simulink model "soc_WLAN_fpga"  (R2024b)
settings: Solver=FixedStepDiscrete  StartTime=0.0  StopTime=stopTime  RelTol=1e-3
PreLoadFcn:
  | addpath(fullfile(matlabroot,'toolbox','whdl','whdlexamples','whdlexamples'));
InitFcn:
  | addpath(fullfile(matlabroot,'toolbox','whdl','whdlexamples','whdlexamples'));
model workspace (MAT data in the model file):
  socvcb : containers.Map (value not decoded)
undefined symbols (not defined in the file): Add, bitRatePerOfdmSym, chanBW, coe, cpLen, dataUpsampleFactor, DelayValMaxNsdMinusLastPilotSc, DescramblerInitialSeed, designMultirateFIR, fftLen, filterLatency, filterUpsampleFactor, Fs, Hd, HT_MFMCS0, HT_MFMCS1, HT_MFMCS2, HT_MFMCS3, HT_MFMCS4, HT_MFMCS5, HT_MFMCS6, HT_MFMCS7, HTUnUsedScInd, inputSamplingRate, interp_coeff, maxPilotRefCounterVale, maxPilotsRef, maxPilotsRefNonHT, Ncol_HT, Ncol_NonHT, noDataSubCarriers, Non_HTMCS0, Non_HTMCS1, Non_HTMCS2, Non_HTMCS3, Non_HTMCS4, Non_HTMCS5, Non_HTMCS6, Non_HTMCS7, Nrow_HT, Nrow_NonHT, numDSC_HT, numDSC_HT_vhtSigB, numDSC_NonHT, numDscHT, numDscNonHT, numOfBitsPerOFDMSym, numOfDataBitsPerOFDMSym, numPilots, numScHT, numSCS_HT, numSCS_NonHT, pnSeq, QAM, rxDownsampleFactor, secondPIdx_HT, secondPIdx_NonHT, Shift, VHTMCS0, VHTMCS1 ... (+7)
libraries: hdlsllib x267, simulink x210, dspsigops x22, whdlutilities x10, whdlmod x9, dsphdlfiltering2 x5, dsphdlmathfun2 x4, whdledac x3, hwlogicconnlib x2, commhdlcrc x2, dsphdlsigops2 x2
(part 5 of 14)

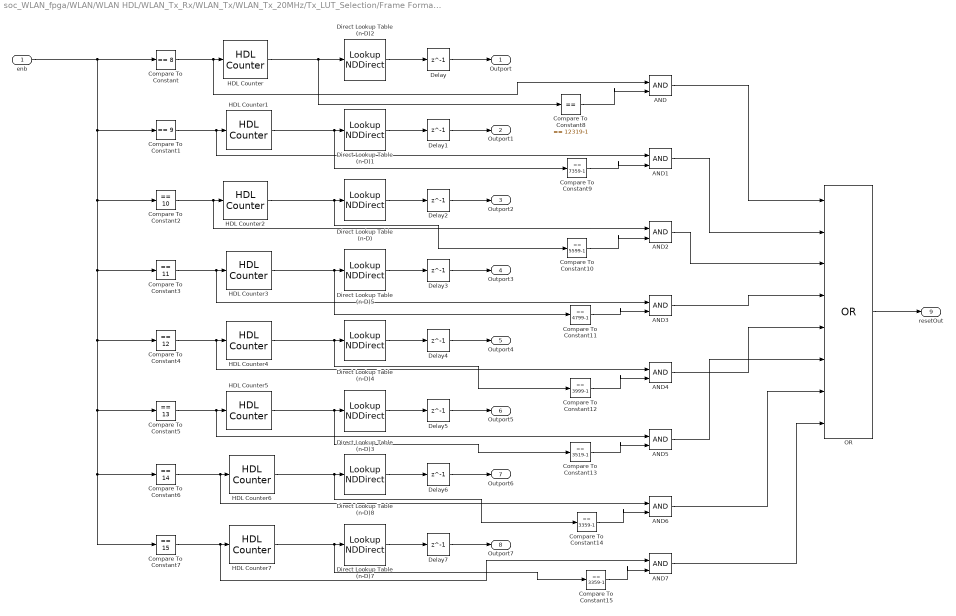
== system soc_WLAN_fpga/WLAN/WLAN HDL/WLAN_Tx_Rx/WLAN_Tx/WLAN_Tx_20MHz/Tx_LUT_Selection/Frame Format 1 ==
  enb : Inport
  AND{,1..7} (8 alike) : Logic  IconShape=distinctive  AllPortsSameDT=off  OutDataTypeStr=boolean
  Compare To Constant : simulink/Logic and Bit Operations/Compare To Constant  relop===  const=8  OutDataTypeStr=boolean
  Compare To Constant1 : simulink/Logic and Bit Operations/Compare To Constant  relop===  const=9  OutDataTypeStr=boolean
  Compare To Constant10 : simulink/Logic and Bit Operations/Compare To Constant  relop===  const=5599-1  OutDataTypeStr=boolean
  Compare To Constant11 : simulink/Logic and Bit Operations/Compare To Constant  relop===  const=4799-1  OutDataTypeStr=boolean
  Compare To Constant12 : simulink/Logic and Bit Operations/Compare To Constant  relop===  const=3999-1  OutDataTypeStr=boolean
  Compare To Constant13 : simulink/Logic and Bit Operations/Compare To Constant  relop===  const=3519-1  OutDataTypeStr=boolean
  Compare To Constant14 : simulink/Logic and Bit Operations/Compare To Constant  relop===  const=3359-1  OutDataTypeStr=boolean
  Compare To Constant15 : simulink/Logic and Bit Operations/Compare To Constant  relop===  const=3359-1  OutDataTypeStr=boolean
  Compare To Constant2 : simulink/Logic and Bit Operations/Compare To Constant  relop===  const=10  OutDataTypeStr=boolean
  Compare To Constant3 : simulink/Logic and Bit Operations/Compare To Constant  relop===  const=11  OutDataTypeStr=boolean
  Compare To Constant4 : simulink/Logic and Bit Operations/Compare To Constant  relop===  const=12  OutDataTypeStr=boolean
  Compare To Constant5 : simulink/Logic and Bit Operations/Compare To Constant  relop===  const=13  OutDataTypeStr=boolean
  Compare To Constant6 : simulink/Logic and Bit Operations/Compare To Constant  relop===  const=14  OutDataTypeStr=boolean
  Compare To Constant7 : simulink/Logic and Bit Operations/Compare To Constant  relop===  const=15  OutDataTypeStr=boolean
  Compare To Constant8 : simulink/Logic and Bit Operations/Compare To Constant  relop===  const=12319-1  OutDataTypeStr=boolean
  Compare To Constant9 : simulink/Logic and Bit Operations/Compare To Constant  relop===  const=7359-1  OutDataTypeStr=boolean
  Delay{,1..7} (8 alike) : Delay  DelayLength=1
  Direct Lookup Table (n-D) : LookupNDDirect  NumberOfTableDimensions=1  Table=HT_MFMCS2
  Direct Lookup Table (n-D)1 : LookupNDDirect  NumberOfTableDimensions=1  Table=HT_MFMCS1
  Direct Lookup Table (n-D)2 : LookupNDDirect  NumberOfTableDimensions=1  Table=HT_MFMCS0
  Direct Lookup Table (n-D)3 : LookupNDDirect  NumberOfTableDimensions=1  Table=HT_MFMCS5
  Direct Lookup Table (n-D)4 : LookupNDDirect  NumberOfTableDimensions=1  Table=HT_MFMCS4
  Direct Lookup Table (n-D)5 : LookupNDDirect  NumberOfTableDimensions=1  Table=HT_MFMCS3
  Direct Lookup Table (n-D)7 : LookupNDDirect  NumberOfTableDimensions=1  Table=HT_MFMCS7
  Direct Lookup Table (n-D)8 : LookupNDDirect  NumberOfTableDimensions=1  Table=HT_MFMCS6
  HDL Counter : hdlsllib/Sources/HDL Counter  CountType=Count limited  CountInit=0  CountStep=1  CountMax=12319  CountFromType=Initial value  CountFrom=0  CountResetPort=off  CountLoadPort=off  CountEnbPort=on  CountDirPort=off  CountHitOutputPort=off  CountDataType=Unsigned  CountWordLen=16  CountFracLen=0  CountSampTime=1
  HDL Counter1 : hdlsllib/Sources/HDL Counter  CountType=Count limited  CountInit=0  CountStep=1  CountMax=7359  CountFromType=Initial value  CountFrom=0  CountResetPort=off  CountLoadPort=off  CountEnbPort=on  CountDirPort=off  CountHitOutputPort=off  CountDataType=Unsigned  CountWordLen=16  CountFracLen=0  CountSampTime=1
  HDL Counter2 : hdlsllib/Sources/HDL Counter  CountType=Count limited  CountInit=0  CountStep=1  CountMax=5599  CountFromType=Initial value  CountFrom=0  CountResetPort=off  CountLoadPort=off  CountEnbPort=on  CountDirPort=off  CountHitOutputPort=off  CountDataType=Unsigned  CountWordLen=16  CountFracLen=0  CountSampTime=1
  HDL Counter3 : hdlsllib/Sources/HDL Counter  CountType=Count limited  CountInit=0  CountStep=1  CountMax=4799  CountFromType=Initial value  CountFrom=0  CountResetPort=off  CountLoadPort=off  CountEnbPort=on  CountDirPort=off  CountHitOutputPort=off  CountDataType=Unsigned  CountWordLen=16  CountFracLen=0  CountSampTime=1
  HDL Counter4 : hdlsllib/Sources/HDL Counter  CountType=Count limited  CountInit=0  CountStep=1  CountMax=3999  CountFromType=Initial value  CountFrom=0  CountResetPort=off  CountLoadPort=off  CountEnbPort=on  CountDirPort=off  CountHitOutputPort=off  CountDataType=Unsigned  CountWordLen=16  CountFracLen=0  CountSampTime=1
  HDL Counter5 : hdlsllib/Sources/HDL Counter  CountType=Count limited  CountInit=0  CountStep=1  CountMax=3519  CountFromType=Initial value  CountFrom=0  CountResetPort=off  CountLoadPort=off  CountEnbPort=on  CountDirPort=off  CountHitOutputPort=off  CountDataType=Unsigned  CountWordLen=16  CountFracLen=0  CountSampTime=1
  HDL Counter6 : hdlsllib/Sources/HDL Counter  CountType=Count limited  CountInit=0  CountStep=1  CountMax=3359  CountFromType=Initial value  CountFrom=0  CountResetPort=off  CountLoadPort=off  CountEnbPort=on  CountDirPort=off  CountHitOutputPort=off  CountDataType=Unsigned  CountWordLen=16  CountFracLen=0  CountSampTime=1
  HDL Counter7 : hdlsllib/Sources/HDL Counter  CountType=Count limited  CountInit=0  CountStep=1  CountMax=3359  CountFromType=Initial value  CountFrom=0  CountResetPort=off  CountLoadPort=off  CountEnbPort=on  CountDirPort=off  CountHitOutputPort=off  CountDataType=Unsigned  CountWordLen=16  CountFracLen=0  CountSampTime=1
  OR : Logic  Operator=OR  Inputs=8  IconShape=distinctive  AllPortsSameDT=off  OutDataTypeStr=boolean
  Outport : Outport
  Outport1 : Outport  Port=2
  Outport2 : Outport  Port=3
  Outport3 : Outport  Port=4
  Outport4 : Outport  Port=5
  Outport5 : Outport  Port=6
  Outport6 : Outport  Port=7
  Outport7 : Outport  Port=8
  resetOut : Outport  Port=9
  wires:
  Delay2/1 -> Outport2/1
  Delay/1 -> Outport/1
  Direct Lookup Table (n-D)1/1 -> Delay1/1
  Direct Lookup Table (n-D)/1 -> Delay2/1
  Direct Lookup Table (n-D)2/1 -> Delay/1
  Delay1/1 -> Outport1/1
  Delay4/1 -> Outport4/1
  Delay5/1 -> Outport5/1
  Direct Lookup Table (n-D)5/1 -> Delay3/1
  Direct Lookup Table (n-D)4/1 -> Delay4/1
  Direct Lookup Table (n-D)3/1 -> Delay5/1
  Delay3/1 -> Outport3/1
  Delay7/1 -> Outport7/1
  Direct Lookup Table (n-D)8/1 -> Delay6/1
  Direct Lookup Table (n-D)7/1 -> Delay7/1
  Delay6/1 -> Outport6/1
  Compare To Constant/1 -> AND/1, HDL Counter/1
  HDL Counter/1 -> Direct Lookup Table (n-D)2/1, Compare To Constant8/1
  HDL Counter1/1 -> Compare To Constant9/1, Direct Lookup Table (n-D)1/1
  Compare To Constant1/1 -> AND1/1, HDL Counter1/1
  HDL Counter2/1 -> Compare To Constant10/1, Direct Lookup Table (n-D)/1
  Compare To Constant2/1 -> AND2/1, HDL Counter2/1
  HDL Counter3/1 -> Compare To Constant11/1, Direct Lookup Table (n-D)5/1
  Compare To Constant3/1 -> AND3/1, HDL Counter3/1
  HDL Counter4/1 -> Compare To Constant12/1, Direct Lookup Table (n-D)4/1
  Compare To Constant4/1 -> AND4/1, HDL Counter4/1
  HDL Counter5/1 -> Compare To Constant13/1, Direct Lookup Table (n-D)3/1
  Compare To Constant5/1 -> AND5/1, HDL Counter5/1
  HDL Counter6/1 -> Compare To Constant14/1, Direct Lookup Table (n-D)8/1
  Compare To Constant6/1 -> AND6/1, HDL Counter6/1
  HDL Counter7/1 -> Compare To Constant15/1, Direct Lookup Table (n-D)7/1
  Compare To Constant7/1 -> AND7/1, HDL Counter7/1
  enb/1 -> Compare To Constant7/1, Compare To Constant6/1, Compare To Constant5/1, Compare To Constant4/1, Compare To Constant3/1, Compare To Constant2/1, Compare To Constant1/1, Compare To Constant/1
  Compare To Constant8/1 -> AND/2
  Compare To Constant9/1 -> AND1/2
  Compare To Constant10/1 -> AND2/2
  Compare To Constant11/1 -> AND3/2
  Compare To Constant12/1 -> AND4/2
  Compare To Constant13/1 -> AND5/2
  Compare To Constant14/1 -> AND6/2
  Compare To Constant15/1 -> AND7/2
  AND/1 -> OR/1
  AND1/1 -> OR/2
  AND2/1 -> OR/3
  AND3/1 -> OR/4
  AND4/1 -> OR/5
  AND5/1 -> OR/6
  AND6/1 -> OR/7
  AND7/1 -> OR/8
  OR/1 -> resetOut/1

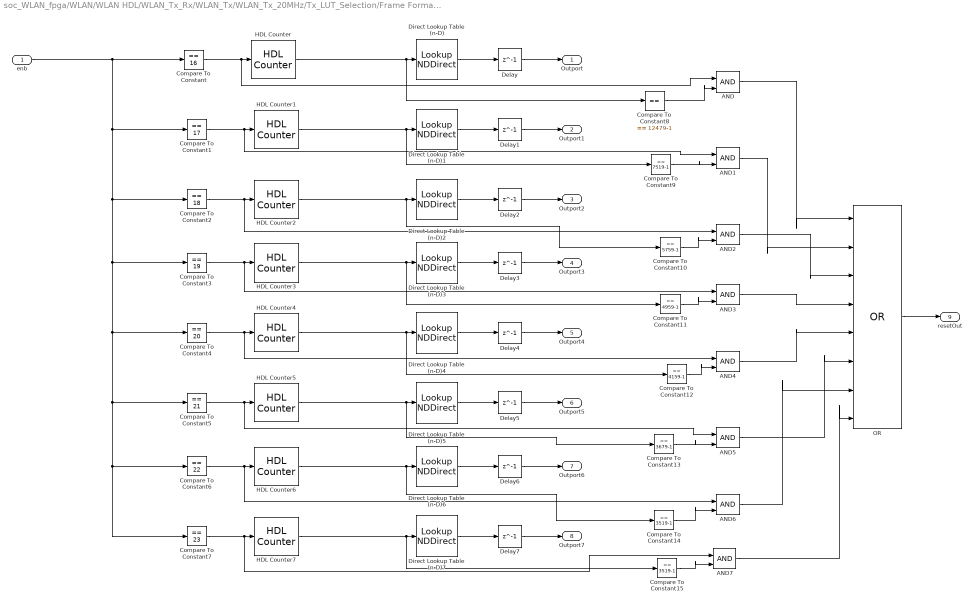
== system soc_WLAN_fpga/WLAN/WLAN HDL/WLAN_Tx_Rx/WLAN_Tx/WLAN_Tx_20MHz/Tx_LUT_Selection/Frame Format 2 ==
  enb : Inport
  AND{,1..7} (8 alike) : Logic  IconShape=distinctive  AllPortsSameDT=off  OutDataTypeStr=boolean
  Compare To Constant : simulink/Logic and Bit Operations/Compare To Constant  relop===  const=16  OutDataTypeStr=boolean
  Compare To Constant1 : simulink/Logic and Bit Operations/Compare To Constant  relop===  const=17  OutDataTypeStr=boolean
  Compare To Constant10 : simulink/Logic and Bit Operations/Compare To Constant  relop===  const=5759-1  OutDataTypeStr=boolean
  Compare To Constant11 : simulink/Logic and Bit Operations/Compare To Constant  relop===  const=4959-1  OutDataTypeStr=boolean
  Compare To Constant12 : simulink/Logic and Bit Operations/Compare To Constant  relop===  const=4159-1  OutDataTypeStr=boolean
  Compare To Constant13 : simulink/Logic and Bit Operations/Compare To Constant  relop===  const=3679-1  OutDataTypeStr=boolean
  Compare To Constant14 : simulink/Logic and Bit Operations/Compare To Constant  relop===  const=3519-1  OutDataTypeStr=boolean
  Compare To Constant15 : simulink/Logic and Bit Operations/Compare To Constant  relop===  const=3519-1  OutDataTypeStr=boolean
  Compare To Constant2 : simulink/Logic and Bit Operations/Compare To Constant  relop===  const=18  OutDataTypeStr=boolean
  Compare To Constant3 : simulink/Logic and Bit Operations/Compare To Constant  relop===  const=19  OutDataTypeStr=boolean
  Compare To Constant4 : simulink/Logic and Bit Operations/Compare To Constant  relop===  const=20  OutDataTypeStr=boolean
  Compare To Constant5 : simulink/Logic and Bit Operations/Compare To Constant  relop===  const=21  OutDataTypeStr=boolean
  Compare To Constant6 : simulink/Logic and Bit Operations/Compare To Constant  relop===  const=22  OutDataTypeStr=boolean
  Compare To Constant7 : simulink/Logic and Bit Operations/Compare To Constant  relop===  const=23  OutDataTypeStr=boolean
  Compare To Constant8 : simulink/Logic and Bit Operations/Compare To Constant  relop===  const=12479-1  OutDataTypeStr=boolean
  Compare To Constant9 : simulink/Logic and Bit Operations/Compare To Constant  relop===  const=7519-1  OutDataTypeStr=boolean
  Delay{,1..7} (8 alike) : Delay  DelayLength=1
  Direct Lookup Table (n-D) : LookupNDDirect  NumberOfTableDimensions=1  Table=VHTMCS0
  Direct Lookup Table (n-D)1 : LookupNDDirect  NumberOfTableDimensions=1  Table=VHTMCS1
  Direct Lookup Table (n-D)2 : LookupNDDirect  NumberOfTableDimensions=1  Table=VHTMCS2
  Direct Lookup Table (n-D)3 : LookupNDDirect  NumberOfTableDimensions=1  Table=VHTMCS3
  Direct Lookup Table (n-D)4 : LookupNDDirect  NumberOfTableDimensions=1  Table=VHTMCS4
  Direct Lookup Table (n-D)5 : LookupNDDirect  NumberOfTableDimensions=1  Table=VHTMCS5
  Direct Lookup Table (n-D)6 : LookupNDDirect  NumberOfTableDimensions=1  Table=VHTMCS6
  Direct Lookup Table (n-D)7 : LookupNDDirect  NumberOfTableDimensions=1  Table=VHTMCS7
  HDL Counter : hdlsllib/Sources/HDL Counter  CountType=Count limited  CountInit=0  CountStep=1  CountMax=12479  CountFromType=Initial value  CountFrom=0  CountResetPort=off  CountLoadPort=off  CountEnbPort=on  CountDirPort=off  CountHitOutputPort=off  CountDataType=Unsigned  CountWordLen=16  CountFracLen=0  CountSampTime=1
  HDL Counter1 : hdlsllib/Sources/HDL Counter  CountType=Count limited  CountInit=0  CountStep=1  CountMax=7519  CountFromType=Initial value  CountFrom=0  CountResetPort=off  CountLoadPort=off  CountEnbPort=on  CountDirPort=off  CountHitOutputPort=off  CountDataType=Unsigned  CountWordLen=16  CountFracLen=0  CountSampTime=1
  HDL Counter2 : hdlsllib/Sources/HDL Counter  CountType=Count limited  CountInit=0  CountStep=1  CountMax=5759  CountFromType=Initial value  CountFrom=0  CountResetPort=off  CountLoadPort=off  CountEnbPort=on  CountDirPort=off  CountHitOutputPort=off  CountDataType=Unsigned  CountWordLen=16  CountFracLen=0  CountSampTime=1
  HDL Counter3 : hdlsllib/Sources/HDL Counter  CountType=Count limited  CountInit=0  CountStep=1  CountMax=4959  CountFromType=Initial value  CountFrom=0  CountResetPort=off  CountLoadPort=off  CountEnbPort=on  CountDirPort=off  CountHitOutputPort=off  CountDataType=Unsigned  CountWordLen=16  CountFracLen=0  CountSampTime=1
  HDL Counter4 : hdlsllib/Sources/HDL Counter  CountType=Count limited  CountInit=0  CountStep=1  CountMax=4159  CountFromType=Initial value  CountFrom=0  CountResetPort=off  CountLoadPort=off  CountEnbPort=on  CountDirPort=off  CountHitOutputPort=off  CountDataType=Unsigned  CountWordLen=16  CountFracLen=0  CountSampTime=1
  HDL Counter5 : hdlsllib/Sources/HDL Counter  CountType=Count limited  CountInit=0  CountStep=1  CountMax=3679  CountFromType=Initial value  CountFrom=0  CountResetPort=off  CountLoadPort=off  CountEnbPort=on  CountDirPort=off  CountHitOutputPort=off  CountDataType=Unsigned  CountWordLen=16  CountFracLen=0  CountSampTime=1
  HDL Counter6 : hdlsllib/Sources/HDL Counter  CountType=Count limited  CountInit=0  CountStep=1  CountMax=3519  CountFromType=Initial value  CountFrom=0  CountResetPort=off  CountLoadPort=off  CountEnbPort=on  CountDirPort=off  CountHitOutputPort=off  CountDataType=Unsigned  CountWordLen=16  CountFracLen=0  CountSampTime=1
  HDL Counter7 : hdlsllib/Sources/HDL Counter  CountType=Count limited  CountInit=0  CountStep=1  CountMax=3519  CountFromType=Initial value  CountFrom=0  CountResetPort=off  CountLoadPort=off  CountEnbPort=on  CountDirPort=off  CountHitOutputPort=off  CountDataType=Unsigned  CountWordLen=16  CountFracLen=0  CountSampTime=1
  OR : Logic  Operator=OR  Inputs=8  IconShape=distinctive  AllPortsSameDT=off  OutDataTypeStr=boolean
  Outport : Outport
  Outport1 : Outport  Port=2
  Outport2 : Outport  Port=3
  Outport3 : Outport  Port=4
  Outport4 : Outport  Port=5
  Outport5 : Outport  Port=6
  Outport6 : Outport  Port=7
  Outport7 : Outport  Port=8
  resetOut : Outport  Port=9
  wires:
  Delay2/1 -> Outport2/1
  Delay/1 -> Outport/1
  Direct Lookup Table (n-D)1/1 -> Delay1/1
  Direct Lookup Table (n-D)2/1 -> Delay2/1
  Direct Lookup Table (n-D)/1 -> Delay/1
  Delay1/1 -> Outport1/1
  Direct Lookup Table (n-D)3/1 -> Delay3/1
  Delay4/1 -> Outport4/1
  Delay3/1 -> Outport3/1
  Delay5/1 -> Outport5/1
  Direct Lookup Table (n-D)5/1 -> Delay5/1
  Direct Lookup Table (n-D)4/1 -> Delay4/1
  Direct Lookup Table (n-D)6/1 -> Delay6/1
  Delay7/1 -> Outport7/1
  Delay6/1 -> Outport6/1
  Direct Lookup Table (n-D)7/1 -> Delay7/1
  Compare To Constant/1 -> AND/1, HDL Counter/1
  HDL Counter/1 -> Compare To Constant8/1, Direct Lookup Table (n-D)/1
  HDL Counter1/1 -> Compare To Constant9/1, Direct Lookup Table (n-D)1/1
  Compare To Constant1/1 -> AND1/1, HDL Counter1/1
  HDL Counter2/1 -> Compare To Constant10/1, Direct Lookup Table (n-D)2/1
  Compare To Constant2/1 -> AND2/1, HDL Counter2/1
  HDL Counter3/1 -> Compare To Constant11/1, Direct Lookup Table (n-D)3/1
  Compare To Constant3/1 -> AND3/1, HDL Counter3/1
  HDL Counter4/1 -> Compare To Constant12/1, Direct Lookup Table (n-D)4/1
  Compare To Constant4/1 -> AND4/1, HDL Counter4/1
  HDL Counter5/1 -> Compare To Constant13/1, Direct Lookup Table (n-D)5/1
  Compare To Constant5/1 -> AND5/1, HDL Counter5/1
  HDL Counter6/1 -> Compare To Constant14/1, Direct Lookup Table (n-D)6/1
  Compare To Constant6/1 -> AND6/1, HDL Counter6/1
  enb/1 -> Compare To Constant7/1, Compare To Constant6/1, Compare To Constant5/1, Compare To Constant4/1, Compare To Constant3/1, Compare To Constant2/1, Compare To Constant1/1, Compare To Constant/1
  HDL Counter7/1 -> Compare To Constant15/1, Direct Lookup Table (n-D)7/1
  Compare To Constant7/1 -> AND7/1, HDL Counter7/1
  Compare To Constant8/1 -> AND/2
  Compare To Constant9/1 -> AND1/2
  Compare To Constant10/1 -> AND2/2
  Compare To Constant11/1 -> AND3/2
  Compare To Constant12/1 -> AND4/2
  Compare To Constant13/1 -> AND5/2
  Compare To Constant14/1 -> AND6/2
  Compare To Constant15/1 -> AND7/2
  AND/1 -> OR/1
  AND1/1 -> OR/2
  AND2/1 -> OR/3
  AND3/1 -> OR/4
  AND4/1 -> OR/5
  AND5/1 -> OR/6
  AND6/1 -> OR/7
  AND7/1 -> OR/8
  OR/1 -> resetOut/1

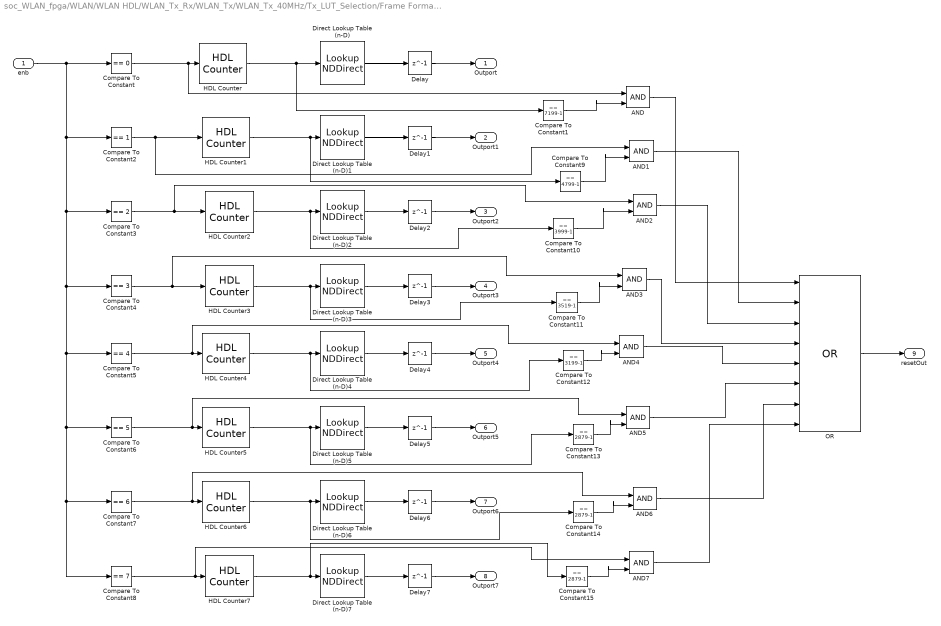
== system soc_WLAN_fpga/WLAN/WLAN HDL/WLAN_Tx_Rx/WLAN_Tx/WLAN_Tx_40MHz/Tx_LUT_Selection/Frame Format 1 ==
  enb : Inport
  AND{,1..7} (8 alike) : Logic  IconShape=distinctive  AllPortsSameDT=off  OutDataTypeStr=boolean
  Compare To Constant : simulink/Logic and Bit Operations/Compare To Constant  relop===  const=0  OutDataTypeStr=boolean
  Compare To Constant1 : simulink/Logic and Bit Operations/Compare To Constant  relop===  const=7199-1  OutDataTypeStr=boolean
  Compare To Constant10 : simulink/Logic and Bit Operations/Compare To Constant  relop===  const=3999-1  OutDataTypeStr=boolean
  Compare To Constant11 : simulink/Logic and Bit Operations/Compare To Constant  relop===  const=3519-1  OutDataTypeStr=boolean
  Compare To Constant12 : simulink/Logic and Bit Operations/Compare To Constant  relop===  const=3199-1  OutDataTypeStr=boolean
  Compare To Constant13 : simulink/Logic and Bit Operations/Compare To Constant  relop===  const=2879-1  OutDataTypeStr=boolean
  Compare To Constant14 : simulink/Logic and Bit Operations/Compare To Constant  relop===  const=2879-1  OutDataTypeStr=boolean
  Compare To Constant15 : simulink/Logic and Bit Operations/Compare To Constant  relop===  const=2879-1  OutDataTypeStr=boolean
  Compare To Constant2 : simulink/Logic and Bit Operations/Compare To Constant  relop===  const=1  OutDataTypeStr=boolean
  Compare To Constant3 : simulink/Logic and Bit Operations/Compare To Constant  relop===  const=2  OutDataTypeStr=boolean
  Compare To Constant4 : simulink/Logic and Bit Operations/Compare To Constant  relop===  const=3  OutDataTypeStr=boolean
  Compare To Constant5 : simulink/Logic and Bit Operations/Compare To Constant  relop===  const=4  OutDataTypeStr=boolean
  Compare To Constant6 : simulink/Logic and Bit Operations/Compare To Constant  relop===  const=5  OutDataTypeStr=boolean
  Compare To Constant7 : simulink/Logic and Bit Operations/Compare To Constant  relop===  const=6  OutDataTypeStr=boolean
  Compare To Constant8 : simulink/Logic and Bit Operations/Compare To Constant  relop===  const=7  OutDataTypeStr=boolean
  Compare To Constant9 : simulink/Logic and Bit Operations/Compare To Constant  relop===  const=4799-1  OutDataTypeStr=boolean
  Delay{,1..7} (8 alike) : Delay  DelayLength=1
  Direct Lookup Table (n-D) : LookupNDDirect  NumberOfTableDimensions=1  Table=HT_MFMCS0
  Direct Lookup Table (n-D)1 : LookupNDDirect  NumberOfTableDimensions=1  Table=HT_MFMCS1
  Direct Lookup Table (n-D)2 : LookupNDDirect  NumberOfTableDimensions=1  Table=HT_MFMCS2
  Direct Lookup Table (n-D)3 : LookupNDDirect  NumberOfTableDimensions=1  Table=HT_MFMCS3
  Direct Lookup Table (n-D)4 : LookupNDDirect  NumberOfTableDimensions=1  Table=HT_MFMCS4
  Direct Lookup Table (n-D)5 : LookupNDDirect  NumberOfTableDimensions=1  Table=HT_MFMCS5
  Direct Lookup Table (n-D)6 : LookupNDDirect  NumberOfTableDimensions=1  Table=HT_MFMCS6
  Direct Lookup Table (n-D)7 : LookupNDDirect  NumberOfTableDimensions=1  Table=HT_MFMCS7
  HDL Counter : hdlsllib/Sources/HDL Counter  CountType=Count limited  CountInit=0  CountStep=1  CountMax=7199  CountFromType=Initial value  CountFrom=0  CountResetPort=off  CountLoadPort=off  CountEnbPort=on  CountDirPort=off  CountHitOutputPort=off  CountDataType=Unsigned  CountWordLen=16  CountFracLen=0  CountSampTime=1
  HDL Counter1 : hdlsllib/Sources/HDL Counter  CountType=Count limited  CountInit=0  CountStep=1  CountMax=4799  CountFromType=Initial value  CountFrom=0  CountResetPort=off  CountLoadPort=off  CountEnbPort=on  CountDirPort=off  CountHitOutputPort=off  CountDataType=Unsigned  CountWordLen=16  CountFracLen=0  CountSampTime=1
  HDL Counter2 : hdlsllib/Sources/HDL Counter  CountType=Count limited  CountInit=0  CountStep=1  CountMax=3999  CountFromType=Initial value  CountFrom=0  CountResetPort=off  CountLoadPort=off  CountEnbPort=on  CountDirPort=off  CountHitOutputPort=off  CountDataType=Unsigned  CountWordLen=16  CountFracLen=0  CountSampTime=1
  HDL Counter3 : hdlsllib/Sources/HDL Counter  CountType=Count limited  CountInit=0  CountStep=1  CountMax=3519  CountFromType=Initial value  CountFrom=0  CountResetPort=off  CountLoadPort=off  CountEnbPort=on  CountDirPort=off  CountHitOutputPort=off  CountDataType=Unsigned  CountWordLen=16  CountFracLen=0  CountSampTime=1
  HDL Counter4 : hdlsllib/Sources/HDL Counter  CountType=Count limited  CountInit=0  CountStep=1  CountMax=3199  CountFromType=Initial value  CountFrom=0  CountResetPort=off  CountLoadPort=off  CountEnbPort=on  CountDirPort=off  CountHitOutputPort=off  CountDataType=Unsigned  CountWordLen=16  CountFracLen=0  CountSampTime=1
  HDL Counter5 : hdlsllib/Sources/HDL Counter  CountType=Count limited  CountInit=0  CountStep=1  CountMax=2879  CountFromType=Initial value  CountFrom=0  CountResetPort=off  CountLoadPort=off  CountEnbPort=on  CountDirPort=off  CountHitOutputPort=off  CountDataType=Unsigned  CountWordLen=16  CountFracLen=0  CountSampTime=1
  HDL Counter6 : hdlsllib/Sources/HDL Counter  CountType=Count limited  CountInit=0  CountStep=1  CountMax=2879  CountFromType=Initial value  CountFrom=0  CountResetPort=off  CountLoadPort=off  CountEnbPort=on  CountDirPort=off  CountHitOutputPort=off  CountDataType=Unsigned  CountWordLen=16  CountFracLen=0  CountSampTime=1
  HDL Counter7 : hdlsllib/Sources/HDL Counter  CountType=Count limited  CountInit=0  CountStep=1  CountMax=2879  CountFromType=Initial value  CountFrom=0  CountResetPort=off  CountLoadPort=off  CountEnbPort=on  CountDirPort=off  CountHitOutputPort=off  CountDataType=Unsigned  CountWordLen=16  CountFracLen=0  CountSampTime=1
  OR : Logic  Operator=OR  Inputs=8  IconShape=distinctive  AllPortsSameDT=off  OutDataTypeStr=boolean
  Outport : Outport
  Outport1 : Outport  Port=2
  Outport2 : Outport  Port=3
  Outport3 : Outport  Port=4
  Outport4 : Outport  Port=5
  Outport5 : Outport  Port=6
  Outport6 : Outport  Port=7
  Outport7 : Outport  Port=8
  resetOut : Outport  Port=9
  wires:
  Direct Lookup Table (n-D)/1 -> Delay/1
  Direct Lookup Table (n-D)1/1 -> Delay1/1
  Direct Lookup Table (n-D)2/1 -> Delay2/1
  Delay/1 -> Outport/1
  Delay1/1 -> Outport1/1
  Delay2/1 -> Outport2/1
  Delay3/1 -> Outport3/1
  Direct Lookup Table (n-D)3/1 -> Delay3/1
  Direct Lookup Table (n-D)5/1 -> Delay5/1
  Direct Lookup Table (n-D)7/1 -> Delay7/1
  Delay4/1 -> Outport4/1
  Direct Lookup Table (n-D)4/1 -> Delay4/1
  Delay7/1 -> Outport7/1
  Delay6/1 -> Outport6/1
  Delay5/1 -> Outport5/1
  Direct Lookup Table (n-D)6/1 -> Delay6/1
  enb/1 -> Compare To Constant/1, Compare To Constant8/1, Compare To Constant7/1, Compare To Constant6/1, Compare To Constant5/1, Compare To Constant4/1, Compare To Constant3/1, Compare To Constant2/1
  Compare To Constant/1 -> AND/1, HDL Counter/1
  HDL Counter/1 -> Direct Lookup Table (n-D)/1, Compare To Constant1/1
  Compare To Constant1/1 -> AND/2
  Compare To Constant2/1 -> AND1/1, HDL Counter1/1
  HDL Counter1/1 -> Compare To Constant9/1, Direct Lookup Table (n-D)1/1
  Compare To Constant3/1 -> HDL Counter2/1, AND2/1
  HDL Counter2/1 -> Compare To Constant10/1, Direct Lookup Table (n-D)2/1
  Compare To Constant4/1 -> HDL Counter3/1, AND3/1
  HDL Counter3/1 -> Compare To Constant11/1, Direct Lookup Table (n-D)3/1
  Compare To Constant5/1 -> AND4/1, HDL Counter4/1
  HDL Counter4/1 -> Compare To Constant12/1, Direct Lookup Table (n-D)4/1
  Compare To Constant6/1 -> AND5/1, HDL Counter5/1
  HDL Counter5/1 -> Compare To Constant13/1, Direct Lookup Table (n-D)5/1
  Compare To Constant7/1 -> AND6/1, HDL Counter6/1
  HDL Counter6/1 -> Compare To Constant14/1, Direct Lookup Table (n-D)6/1
  Compare To Constant8/1 -> AND7/1, HDL Counter7/1
  HDL Counter7/1 -> Compare To Constant15/1, Direct Lookup Table (n-D)7/1
  Compare To Constant9/1 -> AND1/2
  Compare To Constant10/1 -> AND2/2
  Compare To Constant11/1 -> AND3/2
  Compare To Constant12/1 -> AND4/2
  Compare To Constant13/1 -> AND5/2
  Compare To Constant14/1 -> AND6/2
  Compare To Constant15/1 -> AND7/2
  AND/1 -> OR/1
  AND1/1 -> OR/2
  AND2/1 -> OR/3
  AND3/1 -> OR/4
  AND4/1 -> OR/5
  AND5/1 -> OR/6
  AND6/1 -> OR/7
  AND7/1 -> OR/8
  OR/1 -> resetOut/1

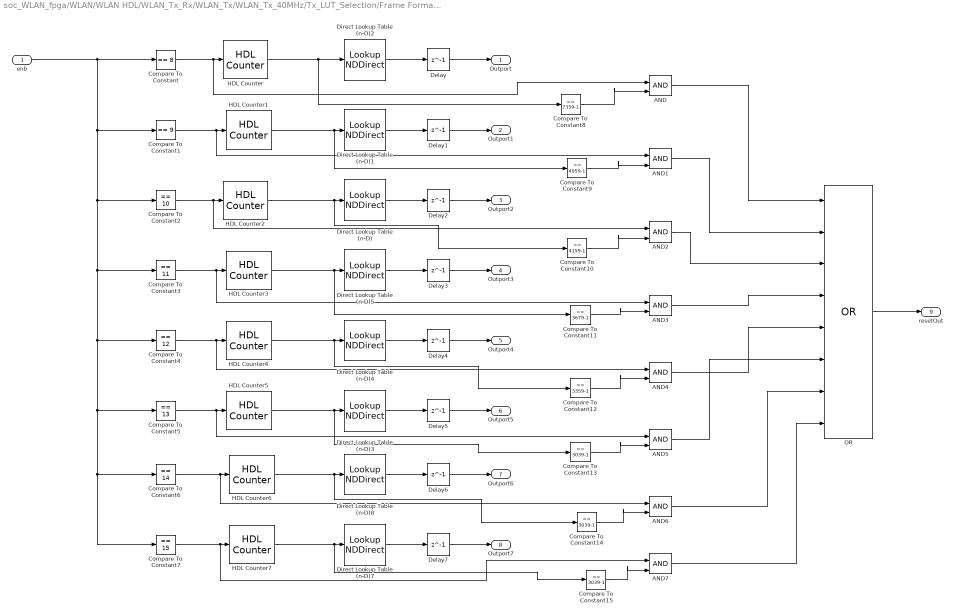
== system soc_WLAN_fpga/WLAN/WLAN HDL/WLAN_Tx_Rx/WLAN_Tx/WLAN_Tx_40MHz/Tx_LUT_Selection/Frame Format 2 ==
  enb : Inport
  AND{,1..7} (8 alike) : Logic  IconShape=distinctive  AllPortsSameDT=off  OutDataTypeStr=boolean
  Compare To Constant : simulink/Logic and Bit Operations/Compare To Constant  relop===  const=8  OutDataTypeStr=boolean
  Compare To Constant1 : simulink/Logic and Bit Operations/Compare To Constant  relop===  const=9  OutDataTypeStr=boolean
  Compare To Constant10 : simulink/Logic and Bit Operations/Compare To Constant  relop===  const=4159-1  OutDataTypeStr=boolean
  Compare To Constant11 : simulink/Logic and Bit Operations/Compare To Constant  relop===  const=3679-1  OutDataTypeStr=boolean
  Compare To Constant12 : simulink/Logic and Bit Operations/Compare To Constant  relop===  const=3359-1  OutDataTypeStr=boolean
  Compare To Constant13 : simulink/Logic and Bit Operations/Compare To Constant  relop===  const=3039-1  OutDataTypeStr=boolean
  Compare To Constant14 : simulink/Logic and Bit Operations/Compare To Constant  relop===  const=3039-1  OutDataTypeStr=boolean
  Compare To Constant15 : simulink/Logic and Bit Operations/Compare To Constant  relop===  const=3039-1  OutDataTypeStr=boolean
  Compare To Constant2 : simulink/Logic and Bit Operations/Compare To Constant  relop===  const=10  OutDataTypeStr=boolean
  Compare To Constant3 : simulink/Logic and Bit Operations/Compare To Constant  relop===  const=11  OutDataTypeStr=boolean
  Compare To Constant4 : simulink/Logic and Bit Operations/Compare To Constant  relop===  const=12  OutDataTypeStr=boolean
  Compare To Constant5 : simulink/Logic and Bit Operations/Compare To Constant  relop===  const=13  OutDataTypeStr=boolean
  Compare To Constant6 : simulink/Logic and Bit Operations/Compare To Constant  relop===  const=14  OutDataTypeStr=boolean
  Compare To Constant7 : simulink/Logic and Bit Operations/Compare To Constant  relop===  const=15  OutDataTypeStr=boolean
  Compare To Constant8 : simulink/Logic and Bit Operations/Compare To Constant  relop===  const=7359-1  OutDataTypeStr=boolean
  Compare To Constant9 : simulink/Logic and Bit Operations/Compare To Constant  relop===  const=4959-1  OutDataTypeStr=boolean
  Delay{,1..7} (8 alike) : Delay  DelayLength=1
  Direct Lookup Table (n-D) : LookupNDDirect  NumberOfTableDimensions=1  Table=VHTMCS2
  Direct Lookup Table (n-D)1 : LookupNDDirect  NumberOfTableDimensions=1  Table=VHTMCS1
  Direct Lookup Table (n-D)2 : LookupNDDirect  NumberOfTableDimensions=1  Table=VHTMCS0
  Direct Lookup Table (n-D)3 : LookupNDDirect  NumberOfTableDimensions=1  Table=VHTMCS5
  Direct Lookup Table (n-D)4 : LookupNDDirect  NumberOfTableDimensions=1  Table=VHTMCS4
  Direct Lookup Table (n-D)5 : LookupNDDirect  NumberOfTableDimensions=1  Table=VHTMCS3
  Direct Lookup Table (n-D)7 : LookupNDDirect  NumberOfTableDimensions=1  Table=VHTMCS7
  Direct Lookup Table (n-D)8 : LookupNDDirect  NumberOfTableDimensions=1  Table=VHTMCS6
  HDL Counter : hdlsllib/Sources/HDL Counter  CountType=Count limited  CountInit=0  CountStep=1  CountMax=7359  CountFromType=Initial value  CountFrom=0  CountResetPort=off  CountLoadPort=off  CountEnbPort=on  CountDirPort=off  CountHitOutputPort=off  CountDataType=Unsigned  CountWordLen=16  CountFracLen=0  CountSampTime=1
  HDL Counter1 : hdlsllib/Sources/HDL Counter  CountType=Count limited  CountInit=0  CountStep=1  CountMax=4959  CountFromType=Initial value  CountFrom=0  CountResetPort=off  CountLoadPort=off  CountEnbPort=on  CountDirPort=off  CountHitOutputPort=off  CountDataType=Unsigned  CountWordLen=16  CountFracLen=0  CountSampTime=1
  HDL Counter2 : hdlsllib/Sources/HDL Counter  CountType=Count limited  CountInit=0  CountStep=1  CountMax=4159  CountFromType=Initial value  CountFrom=0  CountResetPort=off  CountLoadPort=off  CountEnbPort=on  CountDirPort=off  CountHitOutputPort=off  CountDataType=Unsigned  CountWordLen=16  CountFracLen=0  CountSampTime=1
  HDL Counter3 : hdlsllib/Sources/HDL Counter  CountType=Count limited  CountInit=0  CountStep=1  CountMax=3679  CountFromType=Initial value  CountFrom=0  CountResetPort=off  CountLoadPort=off  CountEnbPort=on  CountDirPort=off  CountHitOutputPort=off  CountDataType=Unsigned  CountWordLen=16  CountFracLen=0  CountSampTime=1
  HDL Counter4 : hdlsllib/Sources/HDL Counter  CountType=Count limited  CountInit=0  CountStep=1  CountMax=3359  CountFromType=Initial value  CountFrom=0  CountResetPort=off  CountLoadPort=off  CountEnbPort=on  CountDirPort=off  CountHitOutputPort=off  CountDataType=Unsigned  CountWordLen=16  CountFracLen=0  CountSampTime=1
  HDL Counter5 : hdlsllib/Sources/HDL Counter  CountType=Count limited  CountInit=0  CountStep=1  CountMax=3039  CountFromType=Initial value  CountFrom=0  CountResetPort=off  CountLoadPort=off  CountEnbPort=on  CountDirPort=off  CountHitOutputPort=off  CountDataType=Unsigned  CountWordLen=16  CountFracLen=0  CountSampTime=1
  HDL Counter6 : hdlsllib/Sources/HDL Counter  CountType=Count limited  CountInit=0  CountStep=1  CountMax=3039  CountFromType=Initial value  CountFrom=0  CountResetPort=off  CountLoadPort=off  CountEnbPort=on  CountDirPort=off  CountHitOutputPort=off  CountDataType=Unsigned  CountWordLen=16  CountFracLen=0  CountSampTime=1
  HDL Counter7 : hdlsllib/Sources/HDL Counter  CountType=Count limited  CountInit=0  CountStep=1  CountMax=3039  CountFromType=Initial value  CountFrom=0  CountResetPort=off  CountLoadPort=off  CountEnbPort=on  CountDirPort=off  CountHitOutputPort=off  CountDataType=Unsigned  CountWordLen=16  CountFracLen=0  CountSampTime=1
  OR : Logic  Operator=OR  Inputs=8  IconShape=distinctive  AllPortsSameDT=off  OutDataTypeStr=boolean
  Outport : Outport
  Outport1 : Outport  Port=2
  Outport2 : Outport  Port=3
  Outport3 : Outport  Port=4
  Outport4 : Outport  Port=5
  Outport5 : Outport  Port=6
  Outport6 : Outport  Port=7
  Outport7 : Outport  Port=8
  resetOut : Outport  Port=9
  wires:
  Delay2/1 -> Outport2/1
  Delay/1 -> Outport/1
  Direct Lookup Table (n-D)1/1 -> Delay1/1
  Direct Lookup Table (n-D)/1 -> Delay2/1
  Direct Lookup Table (n-D)2/1 -> Delay/1
  Delay1/1 -> Outport1/1
  Delay4/1 -> Outport4/1
  Delay5/1 -> Outport5/1
  Direct Lookup Table (n-D)5/1 -> Delay3/1
  Direct Lookup Table (n-D)4/1 -> Delay4/1
  Direct Lookup Table (n-D)3/1 -> Delay5/1
  Delay3/1 -> Outport3/1
  Delay7/1 -> Outport7/1
  Direct Lookup Table (n-D)8/1 -> Delay6/1
  Direct Lookup Table (n-D)7/1 -> Delay7/1
  Delay6/1 -> Outport6/1
  Compare To Constant/1 -> AND/1, HDL Counter/1
  HDL Counter/1 -> Direct Lookup Table (n-D)2/1, Compare To Constant8/1
  HDL Counter1/1 -> Compare To Constant9/1, Direct Lookup Table (n-D)1/1
  Compare To Constant1/1 -> AND1/1, HDL Counter1/1
  HDL Counter2/1 -> Compare To Constant10/1, Direct Lookup Table (n-D)/1
  Compare To Constant2/1 -> AND2/1, HDL Counter2/1
  HDL Counter3/1 -> Compare To Constant11/1, Direct Lookup Table (n-D)5/1
  Compare To Constant3/1 -> AND3/1, HDL Counter3/1
  HDL Counter4/1 -> Compare To Constant12/1, Direct Lookup Table (n-D)4/1
  Compare To Constant4/1 -> AND4/1, HDL Counter4/1
  HDL Counter5/1 -> Compare To Constant13/1, Direct Lookup Table (n-D)3/1
  Compare To Constant5/1 -> AND5/1, HDL Counter5/1
  HDL Counter6/1 -> Compare To Constant14/1, Direct Lookup Table (n-D)8/1
  Compare To Constant6/1 -> AND6/1, HDL Counter6/1
  HDL Counter7/1 -> Compare To Constant15/1, Direct Lookup Table (n-D)7/1
  Compare To Constant7/1 -> AND7/1, HDL Counter7/1
  enb/1 -> Compare To Constant7/1, Compare To Constant6/1, Compare To Constant5/1, Compare To Constant4/1, Compare To Constant3/1, Compare To Constant2/1, Compare To Constant1/1, Compare To Constant/1
  Compare To Constant8/1 -> AND/2
  Compare To Constant9/1 -> AND1/2
  Compare To Constant10/1 -> AND2/2
  Compare To Constant11/1 -> AND3/2
  Compare To Constant12/1 -> AND4/2
  Compare To Constant13/1 -> AND5/2
  Compare To Constant14/1 -> AND6/2
  Compare To Constant15/1 -> AND7/2
  AND/1 -> OR/1
  AND1/1 -> OR/2
  AND2/1 -> OR/3
  AND3/1 -> OR/4
  AND4/1 -> OR/5
  AND5/1 -> OR/6
  AND6/1 -> OR/7
  AND7/1 -> OR/8
  OR/1 -> resetOut/1

== system soc_WLAN_fpga/WLAN/WLAN HDL/WLAN_Tx_Rx/WLAN_Rx/WLANHDLReceiver/DataRecovery/Decoder/Depuncturer ==
  dataIn : Inport
  ctrlIn : Inport  Port=2
  codeRate : Inport  Port=3
  vitInputLen : Inport  Port=4
  format : Inport  Port=5
  rstIn : Inport  Port=6
  Delay1 : Delay  DelayLength=5
  Delay13 : Delay
  Delay14 : Delay
  Delay2 : Delay
  Depuncturer1 : Subsystem
  Depuncturer2 : Subsystem
  DepuncturerCtrlGen : Subsystem
  Sample Control Bus Selector : whdlutilities/Sample Control Bus Selector  OutputSignals=start,end,valid
  Switch : Switch  Criteria=u2 > Threshold  SaturateOnIntegerOverflow=off  InputSameDT=off
  Switch1 : Switch  Criteria=u2 > Threshold  SaturateOnIntegerOverflow=off  InputSameDT=off
  Terminator1 : Terminator
  Terminator2 : Terminator
  dataOut : Outport
  ctrl : Outport  Port=2
  wires:
  Sample Control Bus Selector/3 -> Depuncturer2/5(validIn), Depuncturer1/5(validIn), DepuncturerCtrlGen/4(validIn)  "<valid>"
  ctrlIn/1 -> Sample Control Bus Selector/1
  Sample Control Bus Selector/2 -> Terminator2/1  "<end>"
  Sample Control Bus Selector/1 -> Terminator1/1  "<start>"
  Switch/1 -> dataOut/1
  dataIn/1 -> Depuncturer2/1(dataIn), Depuncturer1/1(dataIn)
  rstIn/1 -> DepuncturerCtrlGen/3(rstIn), Depuncturer1/2(rstIn)
  Switch1/1 -> ctrl/1
  Depuncturer2/2(validOut) -> Delay2/1
  Delay13/1 -> Switch/1
  Delay14/1 -> Switch1/2, Switch/2
  Depuncturer1/2(validOut) -> Switch1/3
  Depuncturer1/1(dataOut) -> Switch/3
  codeRate/1 -> Delay1/1, Depuncturer2/3(codeRate)
  Depuncturer2/1(dataOut) -> Delay13/1
  Delay1/1 -> Delay14/1
  Delay2/1 -> Switch1/1
  DepuncturerCtrlGen/2(end) -> Depuncturer2/4(endIn), Depuncturer1/4(endIn)
  DepuncturerCtrlGen/1(start) -> Depuncturer1/3(startIn), Depuncturer2/2(startIn)
  format/1 -> DepuncturerCtrlGen/1(format)
  vitInputLen/1 -> DepuncturerCtrlGen/2(vitInputLen)

== system soc_WLAN_fpga/WLAN/WLAN HDL/WLAN_Tx_Rx/WLAN_Rx/WLANHDLReceiver/DataRecovery/Decoder/ViterbiDecoder ==
  llr : Inport
  validIn : Inport  Port=2
  Data Type Conversion : DataTypeConversion  OutDataTypeStr=int8  SaturateOnIntegerOverflow=off  RndMeth=Floor
  Data Type Conversion1 : DataTypeConversion  OutDataTypeStr=fixdt(1,20,8)  SaturateOnIntegerOverflow=off  RndMeth=Floor
  Gain : Gain  Gain=-1  OutDataTypeStr=Inherit: Same as input
  Shift Arithmetic : ArithShift  BitShiftNumber=4  BitShiftDirection=Left
  Viterbi Decoder : whdledac/Viterbi Decoder  ConstraintLength=7  CodeGenerator=[133 171]  ErasureInputPort=off  Tbd=70  TerminationMethod=Truncated  ResetInputPort=off  SimulateUsing=Code generation
  bit : Outport
  validOut : Outport  Port=2
  wires:
  validIn/1 -> Viterbi Decoder/2
  Viterbi Decoder/2 -> validOut/1
  Viterbi Decoder/1 -> bit/1
  Data Type Conversion/1 -> Gain/1
  llr/1 -> Data Type Conversion1/1
  Gain/1 -> Viterbi Decoder/1
  Data Type Conversion1/1 -> Shift Arithmetic/1
  Shift Arithmetic/1 -> Data Type Conversion/1

== system soc_WLAN_fpga/WLAN/WLAN HDL/WLAN_Tx_Rx/WLAN_Rx/WLANHDLReceiver/DataRecovery/Decoder/vhtSigB ==
  MCS : Inport
  rst : Inport  Port=2
  bit : Inport  Port=3
  ctrlIn : Inport  Port=4
  format : Inport  Port=5
  Delay : Delay  DelayLength=10
  Delay1 : Delay  DelayLength=10
  Delay2 : Delay  DelayLength=10
  Logical Operator : Logic  Operator=NOT  AllPortsSameDT=off  OutDataTypeStr=boolean
  Logical Operator1 : Logic  AllPortsSameDT=off  OutDataTypeStr=boolean
  Logical Operator2 : Logic  AllPortsSameDT=off  OutDataTypeStr=boolean
  Logical Operator3 : Logic  AllPortsSameDT=off  OutDataTypeStr=boolean
  Sample Control Bus Creator : whdlutilities/Sample Control Bus Creator
  Sample Control Bus Selector : whdlutilities/Sample Control Bus Selector  OutputSignals=start,end,valid
  vhtSigBDecoding : Subsystem
  ctrlOut : Outport
  vitInputLen : Outport  Port=2
  psduLen : Outport  Port=3
  vhtCRCRefBits : Outport  Port=4
  vhtCRCRefBitsVld : Outport  Port=5
  wires:
  vhtSigBDecoding/2(psduLen) -> psduLen/1
  bit/1 -> vhtSigBDecoding/3(bit)
  format/1 -> vhtSigBDecoding/4(format)
  MCS/1 -> vhtSigBDecoding/1(MCS)
  Sample Control Bus Selector/2 -> Delay1/1  "<end>"
  ctrlIn/1 -> Sample Control Bus Selector/1
  Sample Control Bus Creator/1 -> ctrlOut/1
  Logical Operator3/1 -> Sample Control Bus Creator/3
  Sample Control Bus Selector/1 -> Delay/1  "<start>"
  vhtSigBDecoding/1(vitInputLen) -> vitInputLen/1
  rst/1 -> vhtSigBDecoding/2(rst)
  Logical Operator2/1 -> Sample Control Bus Creator/2
  Logical Operator1/1 -> Sample Control Bus Creator/1
  vhtSigBDecoding/5(vhtSigBBitVld) -> Logical Operator/1
  Logical Operator/1 -> Logical Operator1/2, Logical Operator2/2, Logical Operator3/2
  Delay/1 -> Logical Operator1/1
  Delay1/1 -> Logical Operator2/1
  Delay2/1 -> Logical Operator3/1
  vhtSigBDecoding/3(vhtCRCRefBits) -> vhtCRCRefBits/1
  vhtSigBDecoding/4(vhtCRCRefBitValid) -> vhtCRCRefBitsVld/1
  Sample Control Bus Selector/3 -> vhtSigBDecoding/5(valid), Delay2/1  "<valid>"

== system soc_WLAN_fpga/WLAN/WLAN HDL/WLAN_Tx_Rx/WLAN_Rx/WLANHDLReceiver/DataRecovery/Deinterleaver/DeInterleaver_HT ==
  wr_din : Inport
  enb : Inport  Port=2
  bps : Inport  Port=3
  rstIn : Inport  Port=4
  numSCs : Inport  Port=5
  Compare To Constant : simulink/Logic and Bit Operations/Compare To Constant  relop=<=  const=numSCS_HT-numPilots-1  OutDataTypeStr=boolean
  Delay : Delay  DelayLength=52  InitialCondition=1
  Delay1 : Delay  DelayLength=1
  Delay2 : Delay  DelayLength=1
  Delay3 : Delay  DelayLength=1  InitialCondition=1
  Delay4 : Delay  DelayLength=52
  Multiport Switch{,1..4} (5 alike) : MultiPortSwitch  Inputs=4  SaturateOnIntegerOverflow=off  InputSameDT=off
  "Stage 2 16QAM " : Subsystem  mask{isInterleaver=off, maxBlkSize=Ncol_HT*Nrow_HT*4, nColumns=Ncol_HT}
      mask prompts: isInterleaver "Interleaver"; maxBlkSize "Maximum block size:"; nColumns "Number of columns:"
      mask init:
      | maxNRows = maxBlkSize/nColumns;
      mask DialogControl ParameterGroupVar Prompt: Interleaver/Deinterleaver
      mask DialogControl Control1 Prompt: Select the Interleaver parameter to use the block as an Interleaver and clear the parameter to use the block as a Deinterleaver.
  Stage 2 64QAM : Subsystem  mask{isInterleaver=off, maxBlkSize=Ncol_HT*Nrow_HT*6, nColumns=Ncol_HT}
      mask prompts: isInterleaver "Interleaver"; maxBlkSize "Maximum block size:"; nColumns "Number of columns:"
      mask init:
      | maxNRows = maxBlkSize/nColumns;
      mask DialogControl ParameterGroupVar Prompt: Interleaver/Deinterleaver
      mask DialogControl Control1 Prompt: Select the Interleaver parameter to use the block as an Interleaver and clear the parameter to use the block as a Deinterleaver.
  Stage 2 BPSK : Subsystem  mask{isInterleaver=off, maxBlkSize=Ncol_HT*Nrow_HT, nColumns=Ncol_HT}
      mask prompts: isInterleaver "Interleaver"; maxBlkSize "Maximum block size:"; nColumns "Number of columns:"
      mask init:
      | maxNRows = maxBlkSize/nColumns;
      mask DialogControl ParameterGroupVar Prompt: Interleaver/Deinterleaver
      mask DialogControl Control1 Prompt: Select the Interleaver parameter to use the block as an Interleaver and clear the parameter to use the block as a Deinterleaver.
  Stage 2 QPSK : Subsystem  mask{isInterleaver=off, maxBlkSize=Ncol_HT*Nrow_HT*2, nColumns=Ncol_HT}
      mask prompts: isInterleaver "Interleaver"; maxBlkSize "Maximum block size:"; nColumns "Number of columns:"
      mask init:
      | maxNRows = maxBlkSize/nColumns;
      mask DialogControl ParameterGroupVar Prompt: Interleaver/Deinterleaver
      mask DialogControl Control1 Prompt: Select the Interleaver parameter to use the block as an Interleaver and clear the parameter to use the block as a Deinterleaver.
  Stage1 : Subsystem
  ctrlGen : Subsystem
  numSCsConverter : Subsystem
  dataOut : Outport
  startOut : Outport  Port=2
  endOut : Outport  Port=3
  validOut : Outport  Port=4
  numSCSFlag : Outport  Port=5
  ready : Outport  Port=6
  wires:
  Stage 2 BPSK/1(dataOut) -> Multiport Switch/2
  bps/1 -> Stage1/3(bps), Delay3/1, numSCsConverter/2(bps)
  wr_din/1 -> Stage1/1(wr_din)
  rstIn/1 -> Delay2/1, Stage1/4(rst)
  enb/1 -> Stage1/2(enb)
  Stage1/1(dataOut) -> Stage 2 BPSK/1(dataIn), Stage 2 QPSK/1(dataIn), "Stage 2 16QAM "/1(dataIn), Stage 2 64QAM/1(dataIn)
  Stage1/2(validOut) -> Stage 2 64QAM/4(validIn), "Stage 2 16QAM "/4(validIn), Stage 2 QPSK/4(validIn), Stage 2 BPSK/4(validIn), ctrlGen/1(enb)
  ctrlGen/1(Out1) -> Stage 2 BPSK/2(startIn), Stage 2 64QAM/2(startIn), "Stage 2 16QAM "/2(startIn), Stage 2 QPSK/2(startIn)
  ctrlGen/2(Out2) -> Stage 2 BPSK/3(endIn), Stage 2 QPSK/3(endIn), "Stage 2 16QAM "/3(endIn), Stage 2 64QAM/3(endIn)
  Stage 2 QPSK/1(dataOut) -> Multiport Switch/3
  "Stage 2 16QAM "/1(dataOut) -> Multiport Switch/4
  Stage 2 64QAM/1(dataOut) -> Multiport Switch/5
  Multiport Switch/1 -> dataOut/1
  Multiport Switch1/1 -> startOut/1
  Multiport Switch2/1 -> endOut/1
  Multiport Switch3/1 -> validOut/1
  Multiport Switch4/1 -> ready/1
  Stage 2 BPSK/3(endOut) -> Multiport Switch2/2
  Stage 2 BPSK/2(startOut) -> Multiport Switch1/2
  Stage 2 QPSK/2(startOut) -> Multiport Switch1/3
  "Stage 2 16QAM "/2(startOut) -> Multiport Switch1/4
  Stage 2 64QAM/2(startOut) -> Multiport Switch1/5
  Stage 2 QPSK/3(endOut) -> Multiport Switch2/3
  "Stage 2 16QAM "/3(endOut) -> Multiport Switch2/4
  Stage 2 64QAM/3(endOut) -> Multiport Switch2/5
  Stage 2 BPSK/4(validOut) -> Multiport Switch3/2
  Stage 2 QPSK/4(validOut) -> Multiport Switch3/3
  "Stage 2 16QAM "/4(validOut) -> Multiport Switch3/4
  Stage 2 64QAM/4(validOut) -> Multiport Switch3/5
  Stage 2 BPSK/5(ready) -> Multiport Switch4/2
  Stage 2 QPSK/5(ready) -> Multiport Switch4/3
  "Stage 2 16QAM "/5(ready) -> Multiport Switch4/4
  Stage 2 64QAM/5(ready) -> Multiport Switch4/5
  numSCsConverter/1(numSCSOut) -> Compare To Constant/1, Stage1/5(numSCs), Delay1/1
  numSCs/1 -> numSCsConverter/1(numSCS)
  Delay2/1 -> ctrlGen/3(rst)
  Delay1/1 -> Delay4/1
  Delay3/1 -> Delay/1
  Compare To Constant/1 -> numSCSFlag/1
  Delay4/1 -> ctrlGen/2(numSCsIn)
  Delay/1 -> Multiport Switch4/1, Multiport Switch3/1, Multiport Switch2/1, Multiport Switch1/1, Multiport Switch/1

== system soc_WLAN_fpga/WLAN/WLAN HDL/WLAN_Tx_Rx/WLAN_Rx/WLANHDLReceiver/DataRecovery/Deinterleaver/DeInterleaver_NonHT ==
  wr_din : Inport
  enb : Inport  Port=2
  bps : Inport  Port=3
  rst : Inport  Port=4
  numSCs : Inport  Port=5
  Delay : Delay  DelayLength=80+75
  Delay1 : Delay  DelayLength=1
  Delay2 : Delay  DelayLength=1
  Delay3 : Delay  DelayLength=1  InitialCondition=1
  Multiport Switch{,1..4} (5 alike) : MultiPortSwitch  Inputs=4  SaturateOnIntegerOverflow=off  InputSameDT=off
  "Stage 2 16QAM " : Subsystem  mask{isInterleaver=off, maxBlkSize=Ncol_NonHT*Nrow_NonHT*4, nColumns=Ncol_NonHT}
      mask prompts: isInterleaver "Interleaver"; maxBlkSize "Maximum block size:"; nColumns "Number of columns:"
      mask init:
      | maxNRows = maxBlkSize/nColumns;
      mask DialogControl ParameterGroupVar Prompt: Interleaver/Deinterleaver
      mask DialogControl Control1 Prompt: Select the Interleaver parameter to use the block as an Interleaver and clear the parameter to use the block as a Deinterleaver.
  Stage 2 64QAM : Subsystem  mask{isInterleaver=off, maxBlkSize=Ncol_NonHT*Nrow_NonHT*6, nColumns=Ncol_NonHT}
      mask prompts: isInterleaver "Interleaver"; maxBlkSize "Maximum block size:"; nColumns "Number of columns:"
      mask init:
      | maxNRows = maxBlkSize/nColumns;
      mask DialogControl ParameterGroupVar Prompt: Interleaver/Deinterleaver
      mask DialogControl Control1 Prompt: Select the Interleaver parameter to use the block as an Interleaver and clear the parameter to use the block as a Deinterleaver.
  Stage 2 BPSK : Subsystem  mask{isInterleaver=off, maxBlkSize=Ncol_NonHT*Nrow_NonHT, nColumns=Ncol_NonHT}
      mask prompts: isInterleaver "Interleaver"; maxBlkSize "Maximum block size:"; nColumns "Number of columns:"
      mask init:
      | maxNRows = maxBlkSize/nColumns;
      mask DialogControl ParameterGroupVar Prompt: Interleaver/Deinterleaver
      mask DialogControl Control1 Prompt: Select the Interleaver parameter to use the block as an Interleaver and clear the parameter to use the block as a Deinterleaver.
  Stage 2 QPSK : Subsystem  mask{isInterleaver=off, maxBlkSize=Ncol_NonHT*Nrow_NonHT*2, nColumns=Ncol_NonHT}
      mask prompts: isInterleaver "Interleaver"; maxBlkSize "Maximum block size:"; nColumns "Number of columns:"
      mask init:
      | maxNRows = maxBlkSize/nColumns;
      mask DialogControl ParameterGroupVar Prompt: Interleaver/Deinterleaver
      mask DialogControl Control1 Prompt: Select the Interleaver parameter to use the block as an Interleaver and clear the parameter to use the block as a Deinterleaver.
  Stage1 : Subsystem
  ctrlGen : Subsystem
  numSCsConverter : Subsystem
  dataOut : Outport
  startOut : Outport  Port=2
  endOut : Outport  Port=3
  validOut : Outport  Port=4
  ready : Outport  Port=5
  wires:
  Stage 2 BPSK/1(dataOut) -> Multiport Switch/2
  bps/1 -> Stage1/3(bps), Delay3/1, numSCsConverter/2(bps)
  wr_din/1 -> Stage1/1(wr_din)
  rst/1 -> Delay/1, Stage1/4(rst)
  enb/1 -> Stage1/2(enb)
  Stage1/1(dataOut) -> Stage 2 BPSK/1(dataIn), Stage 2 QPSK/1(dataIn), "Stage 2 16QAM "/1(dataIn), Stage 2 64QAM/1(dataIn)
  Stage1/2(validOut) -> Stage 2 64QAM/4(validIn), "Stage 2 16QAM "/4(validIn), Stage 2 QPSK/4(validIn), Stage 2 BPSK/4(validIn), ctrlGen/1(enb)
  ctrlGen/1(Out1) -> Stage 2 64QAM/2(startIn), "Stage 2 16QAM "/2(startIn), Stage 2 QPSK/2(startIn), Stage 2 BPSK/2(startIn)
  ctrlGen/2(Out2) -> Stage 2 QPSK/3(endIn), "Stage 2 16QAM "/3(endIn), Stage 2 64QAM/3(endIn), Stage 2 BPSK/3(endIn)
  Stage 2 QPSK/1(dataOut) -> Multiport Switch/3
  "Stage 2 16QAM "/1(dataOut) -> Multiport Switch/4
  Stage 2 64QAM/1(dataOut) -> Multiport Switch/5
  Multiport Switch/1 -> dataOut/1
  Multiport Switch1/1 -> startOut/1
  Multiport Switch2/1 -> endOut/1
  Multiport Switch3/1 -> validOut/1
  Multiport Switch4/1 -> ready/1
  Stage 2 BPSK/3(endOut) -> Multiport Switch2/2
  Stage 2 BPSK/2(startOut) -> Multiport Switch1/2
  Stage 2 QPSK/2(startOut) -> Multiport Switch1/3
  "Stage 2 16QAM "/2(startOut) -> Multiport Switch1/4
  Stage 2 64QAM/2(startOut) -> Multiport Switch1/5
  Stage 2 QPSK/3(endOut) -> Multiport Switch2/3
  "Stage 2 16QAM "/3(endOut) -> Multiport Switch2/4
  Stage 2 64QAM/3(endOut) -> Multiport Switch2/5
  Stage 2 BPSK/4(validOut) -> Multiport Switch3/2
  Stage 2 QPSK/4(validOut) -> Multiport Switch3/3
  "Stage 2 16QAM "/4(validOut) -> Multiport Switch3/4
  Stage 2 64QAM/4(validOut) -> Multiport Switch3/5
  Stage 2 BPSK/5(ready) -> Multiport Switch4/2
  Stage 2 QPSK/5(ready) -> Multiport Switch4/3
  "Stage 2 16QAM "/5(ready) -> Multiport Switch4/4
  Stage 2 64QAM/5(ready) -> Multiport Switch4/5
  numSCsConverter/1(numSCsOut) -> Delay1/1, Stage1/5(numSCs)
  numSCs/1 -> numSCsConverter/1(numSCs)
  Delay/1 -> Delay2/1
  Delay2/1 -> ctrlGen/3(rst)
  Delay1/1 -> ctrlGen/2(numSCs)
  Delay3/1 -> Multiport Switch/1, Multiport Switch1/1, Multiport Switch2/1, Multiport Switch3/1, Multiport Switch4/1
